simulink model "cannon6"  (R2025b)
settings: Solver=VariableStepAuto  StartTime=0.0  StopTime=20.0  RelTol=1e-3
values from neighbouring files (symbols this model uses):
  theta = 35    [cannon_read_to_simulink.m]
settings Model: Creator=Administrator  LastModifiedBy=Administrator

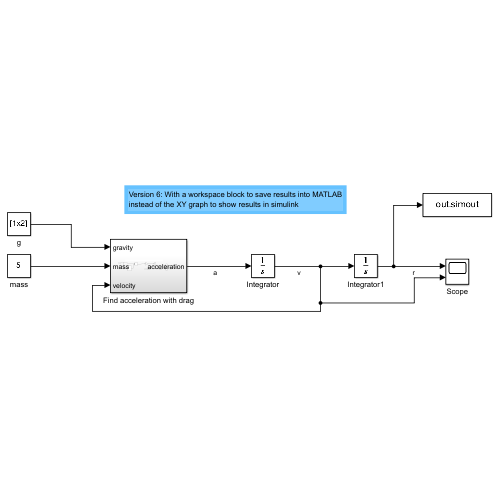
[thumbnail: Simulink's stored preview of the top-level diagram]
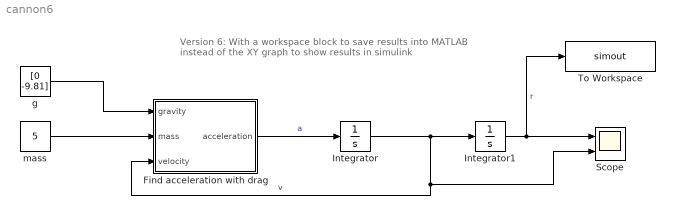
== system cannon6 ==
  note: Version 6: With a workspace block to save results into MATLAB
      | instead of the XY graph to show results in simulink
  Find acceleration with drag : Subsystem
  Integrator : Integrator  InitialCondition=100 * [cosd(theta) sind(theta)]
  Integrator1 : Integrator  InitialCondition=[0 0]
  Scope : Scope  NumInputPorts=2
      settings: ActiveDisplayYMinimum=-447.96370589805508  ActiveDisplayYMaximum=660.11400115553374
  To Workspace : ToWorkspace  VariableName=simout  SaveFormat=Timeseries  SampleTime=-1
  g : Constant  Value=[0 -9.81]
  mass : Constant  Value=5
  wires:
  g/1 -> Find acceleration with drag/1(gravity)
  Integrator/1 -> Scope/2, Find acceleration with drag/3(velocity), Integrator1/1  "v"
  Integrator1/1 -> To Workspace/1, Scope/1  "r"
  mass/1 -> Find acceleration with drag/2(mass)
  Find acceleration with drag/1(acceleration) -> Integrator/1  "a"

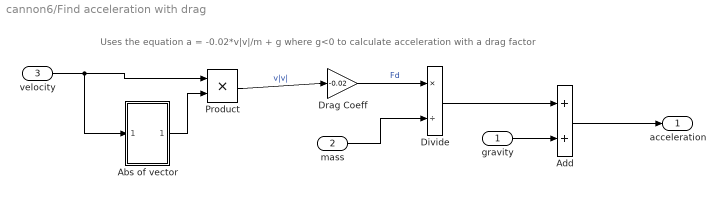
== system cannon6/Find acceleration with drag ==
  note: Uses the equation a = -0.02*v|v|/m + g where g<0 to calculate acceleration with a drag factor
  gravity : Inport
  mass : Inport  Port=2
  velocity : Inport  Port=3
  Abs of vector : Subsystem
  Add : Sum
  Divide : Product  Inputs=*/
  Drag Coeff : Gain  Gain=-0.02
  Product : Product
  acceleration : Outport
  wires:
  velocity/1 -> Abs of vector/1(velocity), Product/1
  Product/1 -> Drag Coeff/1  "v|v|"
  Drag Coeff/1 -> Divide/1  "Fd"
  mass/1 -> Divide/2
  Divide/1 -> Add/1
  gravity/1 -> Add/2
  Add/1 -> acceleration/1
  Abs of vector/1(Out1) -> Product/2

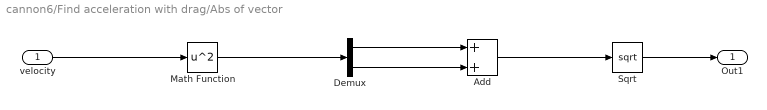
== system cannon6/Find acceleration with drag/Abs of vector ==
  velocity : Inport
  Add : Sum
  Demux : Demux  Outputs=2
  Math Function : Math  Operator=square
  Sqrt : Sqrt
  Out1 : Outport  VectorParamsAs1DForOutWhenUnconnected=off
  wires:
  velocity/1 -> Math Function/1
  Math Function/1 -> Demux/1
  Demux/2 -> Add/2
  Demux/1 -> Add/1
  Add/1 -> Sqrt/1
  Sqrt/1 -> Out1/1
